simulink model "Receiver"  (R2017b)
settings: Solver=FixedStepDiscrete  StartTime=0.0  StopTime=10.0  RelTol=1e-3
InitFcn:
  | modelSettings
undefined symbols (not defined in the file or in its folder): crcDecodeLag, numTrainingSamples, RadioSampleRate, VibertiTracebackLength, xPreambleSeq
libraries: dsphdlfiltering x19, simulink x7, hdlsllib x4, commdigbbndpm3 x2, commcrc2 x1, dspstat3 x1, commseqgen3 x1, commutil2 x1, commcnvcod2 x1
(part 2 of 2)

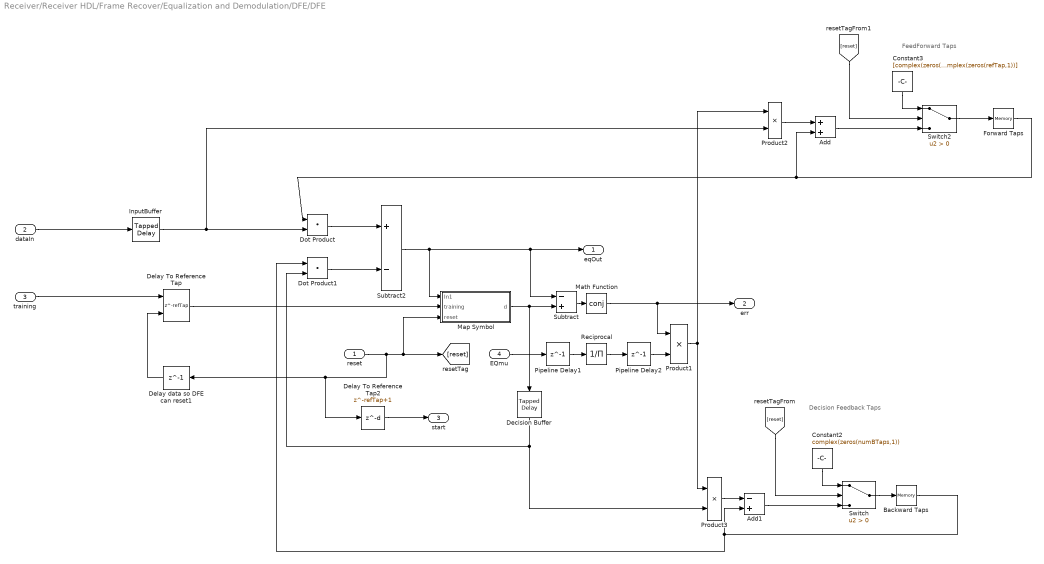
== system Receiver/Receiver HDL/Frame Recover/Equalization and Demodulation/DFE/DFE ==
  note: FeedForward Taps
  note: Decision Feedback Taps
  reset : Inport
  dataIn : Inport  Port=2  OutDataTypeStr=fixdt(1,16,14)
  training : Inport  Port=3  OutDataTypeStr=fixdt(1,16,15)
  EQmu : Inport  Port=4
  Add : Sum  OutDataTypeStr=fixdt(1,16,14)
  Add1 : Sum  Inputs=-+  OutDataTypeStr=fixdt(1,16,19)
  Backward Taps : Memory  InitialCondition=complex(zeros(numBTaps,1))  InheritSampleTime=on
  Constant2 : Constant  Value=complex(zeros(numBTaps,1))  OutDataTypeStr=fixdt(1,16,4)  SampleTime=-1
  Constant3 : Constant  Value=[complex(zeros(numFTaps-1-refTap,1));1;complex(zeros(refTap,1))]  OutDataTypeStr=fixdt(1,16,4)  SampleTime=-1
  Decision Buffer : simulink/Discrete/Tapped Delay  vinit=0.0  samptime=-1  NumDelays=numBTaps  DelayOrder=Oldest  includeCurrent=off
  Delay To Reference Tap : Delay  DelayLength=refTap  ExternalReset=Level
      settings: InputPortMap=u0,r5
  Delay To Reference Tap2 : Delay  DelayLength=refTap+1
  Delay data so DFE can reset1 : Delay  DelayLength=1
  Dot Product : DotProduct  OutDataTypeStr=fixdt(1,16,14)  SaturateOnIntegerOverflow=on  InputSameDT=on
  Dot Product1 : DotProduct  OutDataTypeStr=fixdt(1,16,18)  SaturateOnIntegerOverflow=on  InputSameDT=on
  Forward Taps : Memory  InitialCondition=[complex(zeros(numFTaps-1-refTap,1));1;complex(zeros(refTap,1))]  InheritSampleTime=on
  InputBuffer : simulink/Discrete/Tapped Delay  vinit=0.0  samptime=-1  NumDelays=numFTaps  DelayOrder=Oldest  includeCurrent=off
  Map Symbol : Subsystem
  Math Function : Math  Operator=conj  RndMeth=Zero  SaturateOnIntegerOverflow=on
  Pipeline Delay1 : Delay  DelayLength=1
  Pipeline Delay2 : Delay  DelayLength=1
  Product1 : Product  OutDataTypeStr=fixdt(1,16,22)
  Product2 : Product  OutDataTypeStr=fixdt(1,16,22)
  Product3 : Product  OutDataTypeStr=fixdt(1,16,21)
  Reciprocal : Product  Inputs=/  OutDataTypeStr=fixdt(0,16,22)  SaturateOnIntegerOverflow=on  RndMeth=Zero
  Subtract : Sum  Inputs=-+  OutDataTypeStr=fixdt(1,16,15)
  Subtract2 : Sum  Inputs=+-  OutDataTypeStr=fixdt(1,16,14)
  Switch : Switch  Criteria=u2 > Threshold  OutDataTypeStr=fixdt(1,16,15)
  Switch2 : Switch  Criteria=u2 > Threshold  OutDataTypeStr=fixdt(1,16,14)
  eqOut : Outport
  err : Outport  Port=2
  start : Outport  Port=3
  wires:
  InputBuffer/1 -> Product2/2, Dot Product/2
  Dot Product/1 -> Subtract2/1
  Dot Product1/1 -> Subtract2/2
  Subtract2/1 -> Map Symbol/1(In1), Subtract/1, eqOut/1
  Subtract/1 -> Math Function/1
  Forward Taps/1 -> Dot Product/1, Add/2
  Map Symbol/1(d) -> Subtract/2, Decision Buffer/1
  reset/1 -> Delay To Reference Tap2/1, Delay data so DFE can reset1/1, [reset], Map Symbol/3(reset)
  Backward Taps/1 -> Dot Product1/1, Add1/2
  Decision Buffer/1 -> Product3/2, Dot Product1/2
  Add1/1 -> Switch/3
  Switch/1 -> Backward Taps/1
  Constant2/1 -> Switch/1
  [reset] -> Switch/2
  Switch2/1 -> Forward Taps/1
  Add/1 -> Switch2/3
  Constant3/1 -> Switch2/1
  [reset] -> Switch2/2
  Product2/1 -> Add/1
  Product3/1 -> Add1/1
  dataIn/1 -> InputBuffer/1
  training/1 -> Delay To Reference Tap/1
  Delay To Reference Tap/1 -> Map Symbol/2(training)
  Delay data so DFE can reset1/1 -> Delay To Reference Tap/2
  Delay To Reference Tap2/1 -> start/1
  Reciprocal/1 -> Pipeline Delay2/1
  Pipeline Delay1/1 -> Reciprocal/1
  Pipeline Delay2/1 -> Product1/2
  EQmu/1 -> Pipeline Delay1/1
  Product1/1 -> Product2/1, Product3/1
  Math Function/1 -> err/1, Product1/1

== system Receiver/Receiver HDL/Frame Recover/Equalization and Demodulation/DFE/Packeted To Unpacked ==
  In1 : Inport
  Extract Bits : simulink/Logic and Bit Operations/Extract Bits  bitsToExtract=Range of bits  numBits=8  bitIdxRange=[1]  outScalingMode=Treat bit field as an integer
      settings: SourceProductName=Simulink
  Extract Bits1 : simulink/Logic and Bit Operations/Extract Bits  bitsToExtract=Range of bits  numBits=8  bitIdxRange=[0]  outScalingMode=Treat bit field as an integer
      settings: SourceProductName=Simulink
  Vector Concatenate : Concatenate
  Out1 : Outport
  wires:
  In1/1 -> Extract Bits1/1, Extract Bits/1
  Extract Bits/1 -> Vector Concatenate/1
  Extract Bits1/1 -> Vector Concatenate/2
  Vector Concatenate/1 -> Out1/1

== system Receiver/Receiver HDL/Frame Recover/Equalization and Demodulation/DFE/DFE/Map Symbol ==
  In1 : Inport  OutDataTypeStr=fixdt(1,16,14)
  training : Inport  Port=2  OutDataTypeStr=fixdt(1,16,15)
  reset : Inport  Port=3
  Decision Directed : Subsystem
  Delay : Delay  DelayLength=1
  HDL Counter : hdlsllib/Sources/HDL Counter  CountType=Count limited  CountInit=0  CountStep=1  CountMax=2^18  CountFromType=Initial value  CountFrom=0  CountResetPort=on  CountLoadPort=off  CountEnbPort=off  CountDirPort=off  CountDataType=Unsigned  CountWordLen=32  CountFracLen=0  CountSampTime=1
      settings: SourceProductBaseCode=HD
  Switch : Switch  Criteria=u2 > Threshold  Threshold=numTrainingSamples  OutDataTypeStr=fixdt(1,16,15)
  d : Outport
  wires:
  In1/1 -> Decision Directed/1(eqOut)
  Switch/1 -> d/1
  reset/1 -> HDL Counter/1
  HDL Counter/1 -> Switch/2
  Decision Directed/1(decision) -> Switch/1
  training/1 -> Delay/1
  Delay/1 -> Switch/3

== system Receiver/Receiver HDL/Frame Recover/Equalization and Demodulation/DFE/DFE/Map Symbol/Decision Directed ==
  eqOut : Inport  OutDataTypeStr=fixdt(1,16,14)
  Compare To Zero : simulink/Logic and Bit Operations/Compare To Zero  relop=>=  OutDataTypeStr=boolean
  Compare To Zero1 : simulink/Logic and Bit Operations/Compare To Zero  relop=>=  OutDataTypeStr=boolean
  Complex to Real-Imag : ComplexToRealImag
  QPSK Decisions : LookupNDDirect  Table=[-0.7071 - 0.7071i, -0.7071 + 0.7071i; 0.7071 - 0.7071i, 0.7071 + 0.7071i]  DiagnosticForOutOfRangeInput=Error  TableDataTypeStr=fixdt(1,16,15)
  decision : Outport
  wires:
  eqOut/1 -> Complex to Real-Imag/1
  Complex to Real-Imag/1 -> Compare To Zero/1
  Complex to Real-Imag/2 -> Compare To Zero1/1
  Compare To Zero/1 -> QPSK Decisions/1
  Compare To Zero1/1 -> QPSK Decisions/2
  QPSK Decisions/1 -> decision/1

== matlab function Receiver/Receiver HDL/Viterbi Decode/Buffer/DEBUG: Vitberi Check/MATLAB Function2 ==
  data: bits input; enable input; reset input; crc input
function fcn(bits, enable, reset, crc)
 
persistent buffer index crcEnc crcDec txData

trellis = poly2trellis(7,[171 133]);
tbl = 34;

if isempty(buffer)
    buffer = false(4000,1);
    index = uint16(1);
    ply = 'z^32 + z^26 + z^23 + z^22 + z^16 + z^12 + z^11 + z^10 + z^8 + z^7 + z^5 + z^4 + z^2 + z + 1';
    crcEnc = comm.CRCGenerator('Polynomial',ply);
    crcDec = comm.CRCDetector ('Polynomial',ply);
    rate = 1/2;
    txData = repmat(logical([0;1]), 8*200*log2(4)*rate/2, 1); % Repeating [0 1]
end

if enable
    if reset
       index = uint16(1); 
    end
    
    buffer(index:index+1) = bits;
    index = index + uint16(2);
    if crc%index>3480
        % Generate true data
        crctx = crcEnc(txData);
        dataHardtx = convenc(crctx,trellis);
        % Check
        crcrx = vitdec(buffer(1:3264+tbl*2),trellis,tbl,'cont','hard');
        [rxData,e2] = crcDec(crcrx(tbl+1:tbl+1632));
        % Double check
        crcrx2 = vitdec([dataHardtx;false(tbl*2,1)],trellis,tbl,'cont','hard');
        [rxData2,e2] = crcDec(crcrx2(tbl+1:tbl+1632));
        %[dataHardtx buffer(1:3264)]
        disp(e2);
    end
    if index>4000
        index = uint16(1);
    end
end

== matlab function Receiver/Check Receiver/DMA Capture ==
  data: bytes input; validOut input; sync input; payloadLen input
function fcn(bytes, validOut, sync, payloadLen)

persistent frameBuffer byteCounter fullPayloadBits

bitsInPack = 64;

if isempty(frameBuffer)
    maxFrameBits = (2^16)*8;
    frameBuffer = false(maxFrameBits,1);
    byteCounter = 0;
    fullPayloadBits = uint16(0);
end

if validOut
    if sync
        byteCounter = bitsInPack;
        frameBuffer(1:byteCounter) = bitget(bytes,1:bitsInPack);
        fullPayloadBits = uint16(payloadLen*8);
        
    elseif byteCounter<fullPayloadBits
        frameBuffer(byteCounter+1:byteCounter+bitsInPack) = bitget(bytes,1:bitsInPack);
        byteCounter = byteCounter + bitsInPack;
    else
        if bytes>0
            disp('CRC Error (Outside)');
        else
            disp('Frame passed CRC (Outside)');
        end
    end
end

== matlab function Receiver/Receiver HDL/Viterbi Decode/Buffer/MATLAB Function1 ==
  data: packetLen input; valid input; enablePop output; validOut output; crcStart input; viterbiReset output; crcOut output
function [enablePop,validOut,viterbiReset,crcOut] = manageCurrentDequeue(packetLen, valid, crcStart)

persistent currentBitsInBuffer

bitsPerCycle = uint16(2);
%bitsPerCycleDouble = uint16(4);
viterbiTracebackLengthDouble = uint16(34*2) + uint16(0);

if isempty(currentBitsInBuffer)
    currentBitsInBuffer = uint16(0);
end

if currentBitsInBuffer > viterbiTracebackLengthDouble
    currentBitsInBuffer = currentBitsInBuffer - bitsPerCycle;
    enablePop = true;
    viterbiReset = false;
    crcOut = false;
    validOut = true;
% Trigger packet at length of packet data and let Viterbi eat remaining
% data needed for traceback
elseif currentBitsInBuffer == viterbiTracebackLengthDouble
    currentBitsInBuffer = currentBitsInBuffer - bitsPerCycle;
    enablePop = true;
    viterbiReset = false;
    crcOut = true;
    validOut = false;
% Flush remaining buffered data
elseif (currentBitsInBuffer < viterbiTracebackLengthDouble) &&...
       (currentBitsInBuffer > uint16(0))
    currentBitsInBuffer = currentBitsInBuffer - bitsPerCycle;
    enablePop = true;
    viterbiReset = false;
    crcOut = false;
    validOut = false;
else
    if valid
        if crcStart
            currentBitsInBuffer = packetLen + viterbiTracebackLengthDouble + uint16(0);%bitsPerCycleDouble;
            enablePop = true;
            viterbiReset = true;
            crcOut = false;
            validOut = true;
        else
            enablePop = false;
            viterbiReset = false;
            crcOut = false;
            validOut = false;
        end
    else
        enablePop = false;
        viterbiReset = false;
        crcOut = false;     
        validOut = false;
    end
end

== matlab function Receiver/Receiver HDL/CRC Check and DMA Pack/CRC Check ES/DEBUG: Check CRC Result ==
  data: bits input; start input; done input; valid input; err input
function fcn(bits, start, done, valid, err)

persistent buffer

if isempty(buffer)
    buffer = fi(false(1032,1),0,1,0);
end

buffer = [buffer(2:end);bits];

if done && valid
    if err
        fprintf('CRC Error (HDL CRC)\n');
    else
        fprintf('CRC Passed (HDL CRC)\n');
    end
end
if err % Flag if any error every occurs, if it occurs alone it means given crc is not long enough
    fprintf('CRC Error Type 2 (HDL CRC)\n');
end

== matlab function Receiver/Receiver HDL/CRC Check and DMA Pack/CRC Check ES/DEBUG: CRC Input ==
  data: u input; enable input; endFlag input; startFlag input
function fcn(u, enable,endFlag,startFlag)

persistent buffer crc count
%persistent crcd

if isempty(buffer)
   buffer = false(3000,1); 
    crc = comm.CRCDetector('Polynomial','z^32 + z^26 + z^23 + z^22 + z^16 + z^12 + z^11 + z^10 + z^8 + z^7 + z^5 + z^4 + z^2 + z + 1');
%    crcd = comm.CRCGenerator('Polynomial','z^32 + z^26 + z^23 + z^22 + z^16 + z^12 + z^11 + z^10 + z^8 + z^7 + z^5 + z^4 + z^2 + z + 1');
    count = 1;
end

if enable
    %buffer = [buffer(2:end);u];
    if startFlag
        count = 1;
    elseif count>3000-1
        count = 1;
    else
        count = count + 1;
    end
    buffer(count) = u;
    
    if endFlag
%        disp(count)
        payloadBytes = 8*25;
        k = buffer(1:payloadBytes*8+32);%1632
%         cc = k(end-31:end);
%         front = k(1:64);
%         mid = k(  (65:64+(payloadBytes-2*8)*8) );
%         back = k(end-31-64:end-32);
%         p = crcd(buffer(1:payloadBytes*8));
        [~,e] = crc(k);
        if e
            fprintf('Pre CRC Check Error (at %d)\n',int32(count));
        else
            fprintf('Pre CRC Check Pass (at %d)\n',int32(count));
        end
    end
    
end

== matlab function Receiver/Receiver HDL/Frame Recover/Equalization and Demodulation/2 Bit Descrambler/MATLAB Function ==
  data: bits input; bufferA output; reset input; bufferB output
function [bufferA, bufferB] = BufferSelect(bits,reset)

persistent buffer

% Constants
initBuffer = logical([0 1 0 0 0 1 0]);

% Async
if isempty(buffer)
    buffer = initBuffer;
end

% Reset/Sync
if reset
    bufferA = initBuffer;
    bufferB = [bits(1),initBuffer(1:end-1)];
    buffer = [bits(2),bits(1),initBuffer(1:end-2)];
else
    bufferA = buffer;
    bufferB = [bits(1),buffer(1:end-1)];
    buffer = [bits(2),bits(1),buffer(1:end-2)];    
end

== matlab function Receiver/Receiver HDL/CRC Check and DMA Pack/DMA Interface/Bit Packer ==
  data: bitIn input; byteOut output; startIn input; endIn input; err input; validIn input; validOut output; startOut output
function [byteOut,validOut,startOut] = BitPacker(bitIn, startIn, endIn, err, validIn)

% This block will pack bits into bytes with start boundaries


% Constants
bits2Pack = uint8(64); % byteReg must contain this many bits
zero64 = fi(0,0,64,0);
% NOTE: Frames but be a multiple of bits2Pack or bits will be trimmed from
% end

persistent byteReg byteIndx setStartFlag

if isempty(byteIndx)
    byteReg  = fi(0,0,64,0);
    byteIndx = uint8(1);
    setStartFlag = false;
end

if validIn
    if startIn % Reset
        byteReg = bitset(zero64,1,bitIn);
        byteIndx = uint8(2);
        validOut = false;
        setStartFlag = true;
        startOut = false;
    else
        byteReg = bitset(byteReg,byteIndx,bitIn);
        if byteIndx >= bits2Pack
            byteIndx = uint8(1);
            validOut = true;
            startOut = setStartFlag;
            setStartFlag = false;
        else
            byteIndx = byteIndx + uint8(1);
            validOut = false;
            startOut = false;
        end
    end
elseif endIn % Append error bit to last byte
    byteReg = fi(err,0,64,0);
    validOut = true;
    startOut = false;
else
    validOut = false;
    startOut = false;
end

byteOut = byteReg;

== matlab function Receiver/Receiver HDL/Frame Recover/Enable Equalizer and Packet Decode (Latch) ==
  data: start input; enable output; validIn input
function enable = Counter(start,validIn)

persistent count maxCount lastEOF

if isempty(count)
    count = uint32(0);
    maxCount = uint32(2^16); % Largest possible packet length
    lastEOF = false;
end

eof = false;

if validIn
    % Got a barker preamble start allowing data into equalizer
    if start
        count = maxCount;
    end
    
    % Check on change from true to false
    if lastEOF && ~eof
        %     fprintf('Frame end reached\n');
        count = uint32(0);
    end
    lastEOF = eof;
    
    % Past end of max frame size
    if count>0
        count = count - uint32(1);
    end
    
    % Enable downstream
    enable = count>uint32(0);
else
    enable = false;
end

== matlab function Receiver/Receiver HDL/Frame Recover/Equalization and Demodulation/Subsystem/DEBUG: Header ==
  data: status input; h1 input; h2 input
function HeaderDebug(status,h1,h2)

if status==uint8(2)
    fprintf('Header Check failed (possible false detection)\n');
    fprintf('sum1: %d\n',int32(h1));
    fprintf('sum2: %d\n',int32(h2));
elseif status==uint8(1)
    fprintf('Header Found | Packet is %d bits long\n',int32(h1));
end

== matlab function Receiver/Receiver HDL/Frame Recover/Equalization and Demodulation/DFE/Equalizer ==
  data: trigger input; eqOut output; data input; trainingSymbol input
function eqOut  = dfe(trigger,data,trainingSymbol)

persistent inputBuffer decisionBuffer forwardTaps backwardTaps processedSamples


%% Constants
WL = uint8(16); FL = uint8(14);
F = fimath('SumMode','SpecifyPrecision','SumWordLength',WL,...
    'SumFractionLength',FL);
% Initial delay guess
channelDelay = uint8(0);
% Equalizer settings
mu = fi(0.05,0,10,12);
nFTaps = uint8(11);
nBTaps = uint8(3);
numTrainingSymbols = uint16(250);
resetTaps = fi([complex(zeros(nFTaps-1,1));1],1,WL,FL,F);

%% Async
if isempty(inputBuffer)
    % Set Precisions
    inputBuffer = fi(complex(zeros(nFTaps,1)),1,WL,FL,F);
    decisionBuffer = fi(complex(zeros(nBTaps,1)),1,WL,FL,F);
    forwardTaps = fi(complex(zeros(nFTaps,1)),1,WL,FL,F);
    backwardTaps = fi(complex(zeros(nBTaps,1)),1,WL,FL,F);
    processedSamples = numTrainingSymbols + uint16(1); % Force to DD mode to start
end

%% Reset
if trigger
    processedSamples = uint16(0);
    % Reset taps
    %forwardTaps = fi(complex(zeros(nFTaps,1)),1,WL,FL,F);
    %forwardTaps(nFTaps-channelDelay) = fi(1,1,WL,FL); % Favor specific delay (causes equalizer to converge faster)
    forwardTaps = resetTaps;
    backwardTaps = fi(complex(zeros(nBTaps,1)),1,WL,FL,F);
    % Default output
    eqOut = fi(0,1,WL,FL,F);
else
    %% Equalizer
    % Add data to buffer
    inputBuffer = [inputBuffer(2:end);data];
    
    % Apply equalizer
    eqOut = forwardTaps'*inputBuffer - backwardTaps'*decisionBuffer;
    
    % Determine error
    if (processedSamples<numTrainingSymbols) && (processedSamples>=channelDelay)
        processedSamples = processedSamples + 1;
        d = trainingSymbol;
    else % Decision directed
        % Find closest symbol
        r = real(eqOut)>0; i = imag(eqOut)>0;
        if r
            if i
                d = fi(0.7071 + 0.7071i,1,WL,FL);
            else
                d = fi(0.7071 - 0.7071i,1,WL,FL);
            end
        else
            if i
                d = fi(-0.7071 + 0.7071i,1,WL,FL);
            else
                d = fi(-0.7071 - 0.7071i,1,WL,FL);
            end
        end
    end
    ec = conj(d - eqOut);
    
    % Update taps
    forwardTaps = forwardTaps + mu*ec*inputBuffer;
    backwardTaps = backwardTaps - mu*ec*decisionBuffer;
    
    % Update decision buffer
    db = fi(d,1,WL,FL,F);
    decisionBuffer = [db; decisionBuffer(1:end-1)];
    
end



end

== matlab function Receiver/Receiver HDL/Frame Recover/Equalization and Demodulation/Header Controller ==
  data: enableDownstream output; headerStart input; packetLenBitsOut output; data input; resetViterbi output; crcStart output; status output; s1 output; s2 output
function [enableDownstream,packetLenBitsOut,resetViterbi,crcStart,status,s1,s2] = EvalHeader(headerStart, data)

persistent counter sum1 sum2 packetLenBits lastMode savedPacketLenBits

% The header contains 16 bits, but each bit is duplicated to make checking
% easier
%
% Note this block works on symbols (2bits) but 1 symbol -> 1 decoded bit
%
% PacketLength = (Data+CRC+40(TB)+68)/CodeRate
%
% NOTE TAIL BITS HERE ARE REALLY USED TO DEAL WITH VITERBI LAG SO:
% TailBitsWithLagPadding > TracebackLength

%% Constants
numHeaderBits = uint8(16); % Header is this many bits
powersOfTwo = uint32([1 2 4 8 16 32 64 128 256 512 1024 2048 4096 8192 16384 32768]);
CodeRateINV = uint32(2);%1/CodeRate;
TailBitsWithLagPadding = uint32(uint32(40)+34*2+1); % was +1
% Flag when CRC porition of packet starts relative to header
crcSignalStartLocation = uint32((TailBitsWithLagPadding)*CodeRateINV); % Must be even

% Async
if isempty(counter)
    packetLenBits = uint32(0);
    sum1 = uint32(0);
    sum2 = uint32(0);
    counter = uint8(numHeaderBits);
    lastMode = uint8(3);
    savedPacketLenBits = uint16(0);
end


%% Sync
% Got a header now enable certain mode
if headerStart
    mode = uint8(0);
else
    mode = lastMode;
end

switch mode
    %% Reset on preamble flag and setup for header processing
    case uint8(0)
        crcStart = false;
        resetViterbi = false;
        enableDownstream = false;
        sum1 = uint32(0);
        sum2 = uint32(0);
        counter = uint8(1);
        lastMode = uint8(1); % Go to next state
        packetLenBitsOut = uint16(0);
        status = uint8(0); s1 = uint32(0); s2 = uint32(0);
        
    %% Process header
    case 1 
        crcStart = false;
        enableDownstream = false;
        
        % Convert header bits (bit by bit)
        if data(1)
            sum1 = sum1 + powersOfTwo(counter);
        end
        if data(2)
            sum2 = sum2 + powersOfTwo(counter);
        end
        counter = counter + uint8(1);
        
        if counter>numHeaderBits
            % Check header
            if sum1~=sum2 % Fail
                packetLenBits = uint32(0);
                lastMode = uint8(3);
                resetViterbi = false;
                packetLenBitsOut = uint16(0);
                savedPacketLenBits = uint16(0);
                status = uint8(2); s1 = sum1; s2 = sum2;
            else % Pass
                % Saved header info and trigger downstream
                packetLenBits = uint32(sum1);
                lastMode = uint8(2);
                resetViterbi = true;
                packetLenBitsOut = uint16(sum1-crcSignalStartLocation);
                savedPacketLenBits = uint16(sum1-crcSignalStartLocation);
                status = uint8(1); s1 = sum1; s2 = sum2;
            end
        else
            status = uint8(0); s1 = uint32(0); s2 = uint32(0);
            packetLenBitsOut = uint16(0);
            resetViterbi = false;
        end
        
    %% Decrement sample counter
    case 2 
        status = uint8(0); s1 = uint32(0); s2 = uint32(0);
        resetViterbi = false;
        crcStart = (packetLenBits==crcSignalStartLocation);
        if packetLenBits>uint32(0)
            enableDownstream = true;
            packetLenBits = packetLenBits - uint32(2); % We get 2 bits each call
            packetLenBitsOut = savedPacketLenBits;
        else
            enableDownstream = false;
            lastMode = uint8(3);
            packetLenBitsOut = uint16(0); %Reset
            savedPacketLenBits = uint16(0);%Reset
        end
            
    %% Not processing anything
    otherwise % mode>2
        status = uint8(0); s1 = uint32(0); s2 = uint32(0);
        crcStart = false;
        resetViterbi = false;
        enableDownstream = false;
        packetLenBitsOut = uint16(0);
end

== matlab function Receiver/Receiver HDL/Frame Recover/Frequency Recovery/PED ==
  data: In input; e output
function e  = PED(In)


e = sign(real(In)).*imag(In) - sign(imag(In)).*real(In);

== matlab function Receiver/Receiver HDL/Viterbi Decode/Buffer/MATLAB Function ==
  data: valid input; enable output; start input; crcEnd input
function enable = latch(valid,start,crcEnd)

persistent state

if isempty(state)
    state = false;
end

if start
    enable = true && valid;
    state = true;
elseif crcEnd
    enable = true && valid;
    state = false;
else 
    enable = state && valid;
end
